simulink model "GVCU_HIL_simscape"  (R2026a)
settings: Solver=ode3  StartTime=0  StopTime=10  FixedStep=0.001
model workspace (MAT data in the model file):
  CANoelibParameters : object (value not decoded)
values from neighbouring files (symbols this model uses):
  acc_pedal_data = pedal_data.accelerator_pedal_position_t0    [Init_Simscape_main.m]
  acc_pedal_time = pedal_data.t0    [Init_Simscape_main.m]
  brk_pedal_data = brake_pedal_data.shared_brakes_drvrBrkPedlPerc_t0    [Init_Simscape_main.m]
  brk_pedal_time = brake_pedal_data.t0    [Init_Simscape_main.m]
  cycle_len = zeros(1, num_cycles)    [Init_Simscape_main.m]
  cycle_speed_matrix = zeros(max_cycle_len, num_cycles)    [Init_Simscape_main.m]
  cycle_time_matrix = zeros(max_cycle_len, num_cycles)    [Init_Simscape_main.m]
  veh_speed_data = speed_data.shared_dynamicsVso_vehVelLgt_t0    [Init_Simscape_main.m]
  veh_speed_time = speed_data.t0    [Init_Simscape_main.m]
undefined symbols (not defined in the file or in its folder): Active, aero, AuxActive, bat, brake, config, environment, FL, FL_prs_voltage, FR, FR_prs_voltage, front, pos, powertrain, rear, RL, RL_prs_voltage, RR, RR_prs_voltage, tir, veh, VGetRawValueFlag, Voltage, VT2816_1_Ch1, VT2816_1_Ch2, VT2816_1_Ch3, VT2816_1_Ch4, VT2816_3_Ch13, VT2816_3_Ch14, VT7101_1_Out2, VTS, X, Y, Z
libraries: sm_lib x358, fl_lib x272, nesl_utility x193, canoelib x127, sdl_lib x36, autolibsharedcoupling x21, autolibcoupling x9, slpidlib x7, simulink x3, autolibshareddiff x3, autolibshared x3, autolibutils x1
(part 2 of 17)

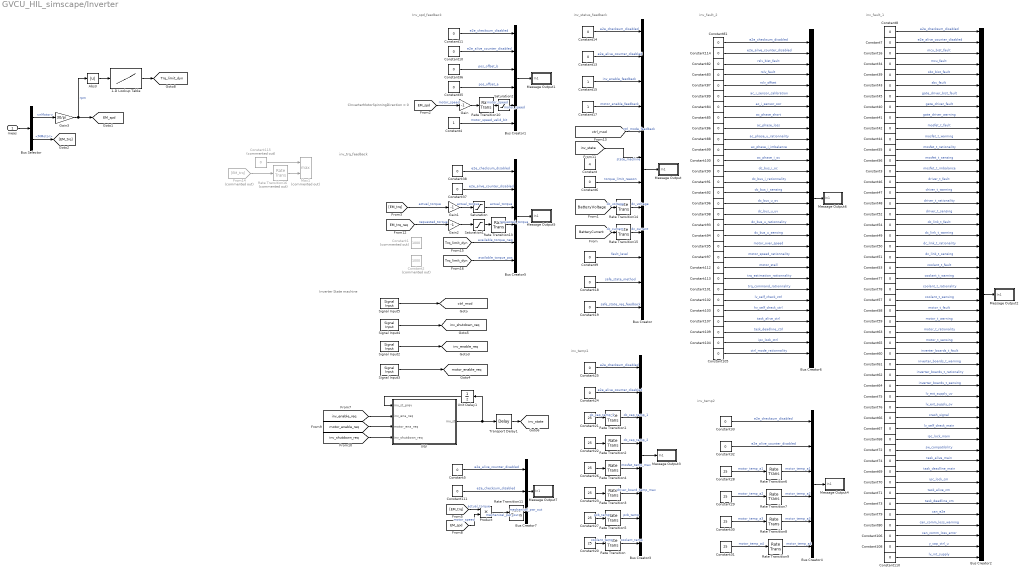
== system GVCU_HIL_simscape/Inverter ==
  note: CInverterMotorSpinningDirection = 0
  note: inv_fault_2
  note: inv_fault_1
  note: inv_trq_feedback
  note: Inv_spd_feedback
  note: Inverter State machine
  note: inv_temp2
  note: inv_temp1
  note: inv_status_feedback
  meas : Inport
  1-D Lookup Table : Lookup_n-D  NumberOfTableDimensions=1  BreakpointsForDimension1=[0, 2000, 3000, 4000, 5000, 6000]  Table=[825, 825, 700, 500, 500, 300]  ExtrapMethod=Clip  UseLastTableValue=on  InternalRulePriority=Speed  RndMeth=Simplest
  Abs3 : Abs  SaturateOnIntegerOverflow=off
  Bus Creator : BusCreator  Inputs=12
  Bus Creator1 : BusCreator  Inputs=6
  Bus Creator2 : BusCreator  Inputs=50
  Bus Creator3 : BusCreator  Inputs=8
  Bus Creator4 : BusCreator  Inputs=6
  Bus Creator5 : BusCreator  Inputs=6
  Bus Creator6 : BusCreator  Inputs=30
  Bus Creator7 : BusCreator  Inputs=3
  Bus Selector : BusSelector  OutputSignals=powertrain.nMotor,powertrain.MMotor
  Constant : Constant  Value=4
  Constant1 : Constant  Commented=on  Value=1000
  Constant{3,5..11,13..14,16,18..19,24..25,32..114} (98 alike) : Constant  Value=0
  Constant115 : Constant  Commented=on  Value=0
  Constant15 : Constant
  Constant17 : Constant
  Constant2 : Constant  Commented=on  Value=1000
  Constant20 : Constant  Value=25  OutDataTypeStr=uint8
  Constant21 : Constant  Value=25  OutDataTypeStr=uint8
  Constant{22..23,26..31} (8 alike) : Constant  Value=25
  Constant4 : Constant
  From14 : From  Commented=on  GotoTag=EM_trq  TagVisibility=global
  Gain : Gain  Gain=-1
  Gain1 : Gain  Gain=-1
  Gain2 : Gain  Gain=-1
  Gain3 : Gain  Gain=30/pi
  INV : MATLAB Function  TreatAsAtomicUnit=on
  Max1 : MinMax  Commented=on  Function=max  Inputs=2
  Message Output : Subsystem  AncestorBlock=canoelib/CANoe I//O/Message Output  mask(Signal Output Module){dbName=inverter_bus, nodeName=INV, msgName=inv_status_feedback, inputType=Bus Signal, rawValue=Default}
      mask prompts: dbName "Database name"; nodeName "Node name"; msgName "Message name"; inputType "Input type"; rawValue "Raw value"
      mask help: Output module for all signals of a databasemessage provided by the CANoe interaction layer. Double click the block for configuration.
      settings: AttributesFormatString=%<msgName>  CopyFcn=set_param(gcb, 'AttributesFormatString', '%<msgName>');  OpenFcn=MessageOutputBlock
      mask Help: For detailed information please refer to the CANoe online help 'MATLAB Integration Package » CANoe I/O Library'.
      mask TypeOptions inputType: Vector | Bus Signal
      mask TypeOptions rawValue: Default | Physical value | Raw value
      mask Display:
      | image(imread('MatlabBlock.png'))
      | disp('CANoe')
  Message Output1 : Subsystem  AncestorBlock=canoelib/CANoe I//O/Message Output  mask(Signal Output Module){dbName=inverter_bus, nodeName=INV, msgName=inv_spd_feedback, inputType=Bus Signal, rawValue=Default}
      mask prompts: dbName "Database name"; nodeName "Node name"; msgName "Message name"; inputType "Input type"; rawValue "Raw value"
      mask help: Output module for all signals of a databasemessage provided by the CANoe interaction layer. Double click the block for configuration.
      settings: AttributesFormatString=%<msgName>  CopyFcn=set_param(gcb, 'AttributesFormatString', '%<msgName>');  OpenFcn=MessageOutputBlock
      mask Help: For detailed information please refer to the CANoe online help 'MATLAB Integration Package » CANoe I/O Library'.
      mask TypeOptions inputType: Vector | Bus Signal
      mask TypeOptions rawValue: Default | Physical value | Raw value
      mask Display:
      | image(imread('MatlabBlock.png'))
      | disp('CANoe')
  Message Output2 : Subsystem  AncestorBlock=canoelib/CANoe I//O/Message Output  mask(Signal Output Module){dbName=inverter_bus, nodeName=INV, msgName=inv_fault_1, inputType=Bus Signal, rawValue=Default}
      mask prompts: dbName "Database name"; nodeName "Node name"; msgName "Message name"; inputType "Input type"; rawValue "Raw value"
      mask help: Output module for all signals of a databasemessage provided by the CANoe interaction layer. Double click the block for configuration.
      settings: AttributesFormatString=inv_fault_1  CopyFcn=set_param(gcb, 'AttributesFormatString', '%<msgName>');  OpenFcn=MessageOutputBlock
      mask Help: For detailed information please refer to the CANoe online help 'MATLAB Integration Package » CANoe I/O Library'.
      mask TypeOptions inputType: Vector | Bus Signal
      mask TypeOptions rawValue: Default | Physical value | Raw value
      mask Display:
      | image(imread('MatlabBlock.png'))
      | disp('CANoe')
  Message Output3 : Subsystem  AncestorBlock=canoelib/CANoe I//O/Message Output  mask(Signal Output Module){dbName=inverter_bus, nodeName=INV, msgName=inv_temperature_1, inputType=Bus Signal, rawValue=Default}
      mask prompts: dbName "Database name"; nodeName "Node name"; msgName "Message name"; inputType "Input type"; rawValue "Raw value"
      mask help: Output module for all signals of a databasemessage provided by the CANoe interaction layer. Double click the block for configuration.
      settings: AttributesFormatString=%<msgName>  CopyFcn=set_param(gcb, 'AttributesFormatString', '%<msgName>');  OpenFcn=MessageOutputBlock
      mask Help: For detailed information please refer to the CANoe online help 'MATLAB Integration Package » CANoe I/O Library'.
      mask TypeOptions inputType: Vector | Bus Signal
      mask TypeOptions rawValue: Default | Physical value | Raw value
      mask Display:
      | image(imread('MatlabBlock.png'))
      | disp('CANoe')
  Message Output4 : Subsystem  AncestorBlock=canoelib/CANoe I//O/Message Output  mask(Signal Output Module){dbName=inverter_bus, nodeName=INV, msgName=inv_temperature_2, inputType=Bus Signal, rawValue=Default}
      mask prompts: dbName "Database name"; nodeName "Node name"; msgName "Message name"; inputType "Input type"; rawValue "Raw value"
      mask help: Output module for all signals of a databasemessage provided by the CANoe interaction layer. Double click the block for configuration.
      settings: AttributesFormatString=%<msgName>  CopyFcn=set_param(gcb, 'AttributesFormatString', '%<msgName>');  OpenFcn=MessageOutputBlock
      mask Help: For detailed information please refer to the CANoe online help 'MATLAB Integration Package » CANoe I/O Library'.
      mask TypeOptions inputType: Vector | Bus Signal
      mask TypeOptions rawValue: Default | Physical value | Raw value
      mask Display:
      | image(imread('MatlabBlock.png'))
      | disp('CANoe')
  Message Output5 : Subsystem  AncestorBlock=canoelib/CANoe I//O/Message Output  mask(Signal Output Module){dbName=inverter_bus, nodeName=INV, msgName=inv_trq_feedback, inputType=Bus Signal, rawValue=Default}
      mask prompts: dbName "Database name"; nodeName "Node name"; msgName "Message name"; inputType "Input type"; rawValue "Raw value"
      mask help: Output module for all signals of a databasemessage provided by the CANoe interaction layer. Double click the block for configuration.
      settings: AttributesFormatString=%<msgName>  CopyFcn=set_param(gcb, 'AttributesFormatString', '%<msgName>');  OpenFcn=MessageOutputBlock
      mask Help: For detailed information please refer to the CANoe online help 'MATLAB Integration Package » CANoe I/O Library'.
      mask TypeOptions inputType: Vector | Bus Signal
      mask TypeOptions rawValue: Default | Physical value | Raw value
      mask Display:
      | image(imread('MatlabBlock.png'))
      | disp('CANoe')
  Message Output6 : Subsystem  AncestorBlock=canoelib/CANoe I//O/Message Output  mask(Signal Output Module){dbName=inverter_bus, nodeName=INV, msgName=inv_fault_2, inputType=Bus Signal, rawValue=Default}
      mask prompts: dbName "Database name"; nodeName "Node name"; msgName "Message name"; inputType "Input type"; rawValue "Raw value"
      mask help: Output module for all signals of a databasemessage provided by the CANoe interaction layer. Double click the block for configuration.
      settings: AttributesFormatString=%<msgName>  CopyFcn=set_param(gcb, 'AttributesFormatString', '%<msgName>');  OpenFcn=MessageOutputBlock
      mask Help: For detailed information please refer to the CANoe online help 'MATLAB Integration Package » CANoe I/O Library'.
      mask TypeOptions inputType: Vector | Bus Signal
      mask TypeOptions rawValue: Default | Physical value | Raw value
      mask Display:
      | image(imread('MatlabBlock.png'))
      | disp('CANoe')
  Message Output7 : Subsystem  AncestorBlock=canoelib/CANoe I//O/Message Output  mask(Signal Output Module){dbName=inverter_bus, nodeName=INV, msgName=inv_pwr_feedback, inputType=Bus Signal, rawValue=Default}
      mask prompts: dbName "Database name"; nodeName "Node name"; msgName "Message name"; inputType "Input type"; rawValue "Raw value"
      mask help: Output module for all signals of a databasemessage provided by the CANoe interaction layer. Double click the block for configuration.
      settings: AttributesFormatString=%<msgName>  CopyFcn=set_param(gcb, 'AttributesFormatString', '%<msgName>');  OpenFcn=MessageOutputBlock
      mask Help: For detailed information please refer to the CANoe online help 'MATLAB Integration Package » CANoe I/O Library'.
      mask TypeOptions inputType: Vector | Bus Signal
      mask TypeOptions rawValue: Default | Physical value | Raw value
      mask Display:
      | image(imread('MatlabBlock.png'))
      | disp('CANoe')
  Product : Product
  Rate Transition{,1..9} (10 alike) : RateTransition  OutPortSampleTime=1
  Rate Transition10 : RateTransition  OutPortSampleTime=0.004
  Rate Transition11 : RateTransition  OutPortSampleTime=0.004
  Rate Transition13 : RateTransition  OutPortSampleTime=0.004
  Rate Transition14 : RateTransition  OutPortSampleTime=0.1
  Rate Transition15 : RateTransition  OutPortSampleTime=0.1
  Rate Transition16 : RateTransition  Commented=on  OutPortSampleTime=0.005
  Saturation : Saturate  UpperLimit=2047  LowerLimit=-2048
  Saturation1 : Saturate  UpperLimit=2047  LowerLimit=-2048
  Saturation2 : Saturate  UpperLimit=16383  LowerLimit=-16384
  Signal Input2 : canoelib/CANoe I//O/Signal Input  dbName=inverter_bus  nodeName=GVCU  msgName=inv_cmd  sigName=inv_enable_req  editSampleTime=0  rawValue=Default  dataType=Default  dataTypeDB=boolean  hasEncoding=off
      settings: AttributesFormatString=%<sigName>  SourceProductName=Vector CANoe
  Signal Input3 : canoelib/CANoe I//O/Signal Input  dbName=inverter_bus  nodeName=GVCU  msgName=inv_cmd  sigName=motor_enable_req  editSampleTime=0  rawValue=Default  dataType=Default  dataTypeDB=boolean  hasEncoding=off
      settings: AttributesFormatString=%<sigName>  SourceProductName=Vector CANoe
  Signal Input4 : canoelib/CANoe I//O/Signal Input  dbName=inverter_bus  nodeName=GVCU  msgName=inv_cmd  sigName=shutdown_req  editSampleTime=0  rawValue=Default  dataType=Default  dataTypeDB=boolean  hasEncoding=off
      settings: AttributesFormatString=%<sigName>  SourceProductName=Vector CANoe
  Signal Input5 : canoelib/CANoe I//O/Signal Input  dbName=inverter_bus  nodeName=GVCU  msgName=inv_cmd  sigName=ctrl_mode_req  editSampleTime=0  rawValue=Default  dataType=Default  dataTypeDB=uint8  hasEncoding=off
      settings: AttributesFormatString=%<sigName>  SourceProductName=Vector CANoe
  Transport Delay1 : TransportDelay
  Unit Delay1 : UnitDelay  SampleTime=-1
  tag scope: EM_spd=global, Trq_limit_dyn=global, ctrl_mod=global, inv_enable_req=global, inv_shutdown_req=global, inv_state=global, motor_enable_req=global
  wires:
  [Trq_limit_dyn] -> Bus Creator5/5  "available_torque_neg"
  [Trq_limit_dyn] -> Bus Creator5/6  "available_torque_pos"
  [EM_trq] -> Gain1/1  "actual_torque"
  Constant4/1 -> Bus Creator1/6  "motor_speed_valid_bit"
  Rate Transition10/1 -> Saturation2/1  "motor_speed"
  Constant6/1 -> Bus Creator/7  "torque_limit_reason"
  Constant10/1 -> Bus Creator1/2  "e2e_alive_counter_disabled"
  Constant11/1 -> Bus Creator1/1  "e2e_checksum_disabled"
  Rate Transition15/1 -> Bus Creator/9  "dc_current"
  Rate Transition14/1 -> Bus Creator/8  "dc_voltage"
  Rate Transition/1 -> Bus Creator3/8  "coolant_temp"
  Rate Transition1/1 -> Bus Creator3/3  "dc_cap_temp_1"
  Rate Transition3/1 -> Bus Creator3/6  "driver_board_temp_max"
  Rate Transition2/1 -> Bus Creator3/4  "dc_cap_temp_2"
  Constant24/1 -> Bus Creator3/2  "e2e_alive_counter_disabled"
  Constant25/1 -> Bus Creator3/1  "e2e_checksum_disabled"
  Rate Transition4/1 -> Bus Creator3/5  "mosfet_temp_max"
  Rate Transition5/1 -> Bus Creator3/7  "pcb_temp"
  Rate Transition6/1 -> Bus Creator4/3  "motor_temp_a1"
  Rate Transition7/1 -> Bus Creator4/4  "motor_temp_a2"
  Rate Transition8/1 -> Bus Creator4/5  "motor_temp_a3"
  Rate Transition9/1 -> Bus Creator4/6  "motor_temp_a4"
  Constant32/1 -> Bus Creator4/2  "e2e_alive_counter_disabled"
  Constant33/1 -> Bus Creator4/1  "e2e_checksum_disabled"
  Signal Input2/1 -> [inv_enable_req]
  Signal Input3/1 -> [motor_enable_req]
  Signal Input4/1 -> [inv_shutdown_req]
  [inv_enable_req] -> INV/2(inv_ena_req)
  [motor_enable_req] -> INV/3(motor_ena_req)
  [inv_shutdown_req] -> INV/4(inv_shutdown_req)
  INV/1(inv_st) -> Unit Delay1/1, Transport Delay1/1
  Transport Delay1/1 -> [inv_state]
  Unit Delay1/1 -> INV/1(inv_st_prev)
  Bus Creator/1 -> Message Output/1(In1)
  Bus Creator3/1 -> Message Output3/1(In1)
  Bus Creator4/1 -> Message Output4/1(In1)
  Constant35/1 -> Bus Creator1/4  "pos_offset_a"
  Constant36/1 -> Bus Creator1/3  "pos_offset_b"
  Bus Creator1/1 -> Message Output1/1(In1)
  Constant37/1 -> Bus Creator5/2  "e2e_alive_counter_disabled"
  Constant38/1 -> Bus Creator5/1  "e2e_checksum_disabled"
  Rate Transition13/1 -> Bus Creator5/4  "requested_torque"
  Bus Creator5/1 -> Message Output5/1(In1)
  Constant18/1 -> Bus Creator/11  "safe_state_method"
  Constant19/1 -> Bus Creator/12  "safe_state_req_feedback"
  Constant14/1 -> Bus Creator/1  "e2e_checksum_disabled"
  Constant13/1 -> Bus Creator/2  "e2e_alive_counter_disabled"
  [inv_state] -> Bus Creator/6  "state_machine"
  [ctrl_mod] -> Bus Creator/5  "ctrl_mode_feedback"
  Constant17/1 -> Bus Creator/4  "motor_enable_feedback"
  Constant15/1 -> Bus Creator/3  "inv_enable_feedback"
  Constant9/1 -> Bus Creator/10  "fault_level"
  Constant7/1 -> Bus Creator2/2  "e2e_alive_counter_disabled"
  Constant8/1 -> Bus Creator2/1  "e2e_checksum_disabled"
  Constant16/1 -> Bus Creator2/3  "mcu_bist_fault"
  Constant40/1 -> Bus Creator2/8  "gate_driver_fault"
  Constant45/1 -> Bus Creator2/7  "gate_driver_bist_fault"
  Constant54/1 -> Bus Creator2/19  "dc_link_t_fault"
  Constant46/1 -> Bus Creator2/15  "driver_t_fault"
  Constant56/1 -> Bus Creator2/13  "mosfet_t_sensing"
  Constant55/1 -> Bus Creator2/12  "mosfet_t_rationality"
  Constant34/1 -> Bus Creator2/4  "mcu_fault"
  Constant39/1 -> Bus Creator2/5  "sbc_bist_fault"
  Constant43/1 -> Bus Creator2/6  "sbc_fault"
  Constant41/1 -> Bus Creator2/9  "gate_driver_warning"
  Constant42/1 -> Bus Creator2/10  "mosfet_t_fault"
  Constant44/1 -> Bus Creator2/11  "mosfet_t_warning"
  Constant47/1 -> Bus Creator2/16  "driver_t_warning"
  Constant48/1 -> Bus Creator2/17  "driver_t_rationality"
  Constant52/1 -> Bus Creator2/18  "driver_t_sensing"
  Constant49/1 -> Bus Creator2/20  "dc_link_t_warning"
  Constant50/1 -> Bus Creator2/21  "dc_link_t_rationality"
  Constant51/1 -> Bus Creator2/22  "dc_link_t_sensing"
  Constant53/1 -> Bus Creator2/23  "coolant_t_fault"
  Constant77/1 -> Bus Creator2/24  "coolant_t_warning"
  Constant78/1 -> Bus Creator2/25  "coolant_t_rationality"
  Constant57/1 -> Bus Creator2/26  "coolant_t_sensing"
  Constant58/1 -> Bus Creator2/27  "motor_t_fault"
  Constant59/1 -> Bus Creator2/28  "motor_t_warning"
  Constant63/1 -> Bus Creator2/29  "motor_t_rationality"
  Constant65/1 -> Bus Creator2/30  "motor_t_sensing"
  Constant60/1 -> Bus Creator2/31  "inverter_boards_t_fault"
  Constant61/1 -> Bus Creator2/32  "inverter_boards_t_warning"
  Constant62/1 -> Bus Creator2/33  "inverter_boards_t_rationality"
  Constant64/1 -> Bus Creator2/34  "inverter_boards_t_sensing"
  Constant75/1 -> Bus Creator2/35  "lv_ext_supply_uv"
  Constant76/1 -> Bus Creator2/36  "lv_ext_supply_ov"
  Constant66/1 -> Bus Creator2/37  "crash_signal"
  Constant67/1 -> Bus Creator2/38  "lv_self_check_main"
  Constant68/1 -> Bus Creator2/39  "ipc_lock_main"
  Constant72/1 -> Bus Creator2/40  "sw_compatibility"
  Constant74/1 -> Bus Creator2/41  "task_alive_main"
  Constant69/1 -> Bus Creator2/42  "task_deadline_main"
  Constant70/1 -> Bus Creator2/43  "ipc_lock_cm"
  Constant71/1 -> Bus Creator2/44  "task_alive_cm"
  Constant73/1 -> Bus Creator2/45  "task_deadline_cm"
  Constant80/1 -> Bus Creator2/47  "can_comm_loss_warning"
  Constant79/1 -> Bus Creator2/46  "can_e2e"
  Bus Creator2/1 -> Message Output2/1(In1)
  Constant86/1 -> Bus Creator6/9  "ac_phase_loss"
  Constant85/1 -> Bus Creator6/8  "ac_phase_short"
  Constant84/1 -> Bus Creator6/7  "ac_i_sensor_oor"
  Constant89/1 -> Bus Creator6/6  "ac_i_sensor_calibration"
  Constant83/1 -> Bus Creator6/4  "rslv_fault"
  Constant87/1 -> Bus Creator6/5  "rslv_offset"
  Constant82/1 -> Bus Creator6/3  "rslv_bist_fault"
  Constant81/1 -> Bus Creator6/1  "e2e_checksum_disabled"
  Constant114/1 -> Bus Creator6/2  "e2e_alive_counter_disabled"
  Constant88/1 -> Bus Creator6/10  "ac_phase_u_rationnality"
  Constant99/1 -> Bus Creator6/11  "ac_phase_i_imbalance"
  Constant100/1 -> Bus Creator6/12  "ac_phase_i_oc"
  Constant90/1 -> Bus Creator6/13  "dc_bus_i_oc"
  Constant91/1 -> Bus Creator6/14  "dc_bus_i_rationnality"
  Constant92/1 -> Bus Creator6/15  "dc_bus_i_sensing"
  Constant96/1 -> Bus Creator6/16  "dc_bus_u_ov"
  Constant98/1 -> Bus Creator6/17  "dc_bus_u_uv"
  Constant93/1 -> Bus Creator6/18  "dc_bus_u_rationnality"
  Constant94/1 -> Bus Creator6/19  "dc_bus_u_sensing"
  Constant95/1 -> Bus Creator6/20  "motor_over_speed"
  Constant97/1 -> Bus Creator6/21  "motor_speed_rationnality"
  Constant112/1 -> Bus Creator6/22  "motor_stall"
  Constant113/1 -> Bus Creator6/23  "trq_estimation_rationnality"
  Constant101/1 -> Bus Creator6/24  "trq_command_rationnality"
  Constant102/1 -> Bus Creator6/25  "lv_self_check_ctrl"
  Constant103/1 -> Bus Creator6/26  "hv_self_check_ctrl"
  Constant107/1 -> Bus Creator6/27  "task_alive_ctrl"
  Constant109/1 -> Bus Creator6/28  "task_deadline_ctrl"
  Constant104/1 -> Bus Creator6/29  "ipc_lock_ctrl"
  Constant105/1 -> Bus Creator6/30  "ctrl_mode_rationnality"
  Bus Creator6/1 -> Message Output6/1(In1)
  Constant106/1 -> Bus Creator2/48  "can_comm_loss_error"
  Constant108/1 -> Bus Creator2/49  "y_cap_ctrl_u"
  Constant110/1 -> Bus Creator2/50  "lv_int_supply"
  Constant20/1 -> Rate Transition/1  "coolant_temp"
  Constant21/1 -> Rate Transition1/1  "dc_cap_temp_1"
  Constant22/1 -> Rate Transition2/1
  Constant23/1 -> Rate Transition3/1
  Constant26/1 -> Rate Transition4/1
  Constant27/1 -> Rate Transition5/1  "pcb_temp"
  Constant28/1 -> Rate Transition6/1  "motor_temp_a1"
  Constant29/1 -> Rate Transition7/1  "motor_temp_a2"
  Constant30/1 -> Rate Transition8/1  "motor_temp_a3"
  Constant31/1 -> Rate Transition9/1  "motor_temp_a4"
  [EM_trq] -> Product/1  "actual_torque"
  [EM_spd] -> Product/2  "motor_speed"
  Rate Transition11/1 -> Bus Creator7/3  "mechanical_pwr_out"
  Constant111/1 -> Bus Creator7/2  "e2e_checksum_disabled"
  Constant5/1 -> Bus Creator7/1  "e2e_alive_counter_disabled"
  Bus Creator7/1 -> Message Output7/1(In1)
  [EM_spd] -> Gain/1  "motor_speed"
  [EM_trq_req] -> Gain2/1  "requested_torque"
  Product/1 -> Rate Transition11/1  "mechanical_pwr_out"
  [BatteryVoltage] -> Rate Transition14/1  "dc_voltage"
  [BatteryCurrent] -> Rate Transition15/1  "dc_current"
  Signal Input5/1 -> [ctrl_mod]
  Constant3/1 -> Bus Creator2/14  "mosfet_t_imbalance"
  Gain/1 -> Rate Transition10/1
  Gain1/1 -> Saturation/1  "actual_torque"
  Gain2/1 -> Saturation1/1
  Constant115/1 -> Max1/1
  Rate Transition16/1 -> Max1/2
  From14/1 -> Rate Transition16/1
  Saturation/1 -> Bus Creator5/3  "actual_torque"
  Saturation1/1 -> Rate Transition13/1
  Saturation2/1 -> Bus Creator1/5  "motor_speed"
  meas/1 -> Bus Selector/1
  Bus Selector/2 -> [EM_trq]  "<MMotor>"
  Bus Selector/1 -> Gain3/1  "<nMotor>"
  1-D Lookup Table/1 -> [Trq_limit_dyn]
  Gain3/1 -> Abs3/1, [EM_spd]  "rpm"
  Abs3/1 -> 1-D Lookup Table/1

== system GVCU_HIL_simscape/Model_observation ==
  note: Vehicle model
  note: Powertrain model
  note: Front axle model
  note: Driver model
  note: AWD Powertrain model
  From10 : From  Commented=on  GotoTag=FR_R_Spd  TagVisibility=global
  From11 : From  Commented=on  GotoTag=FR_G_Spd  TagVisibility=global
  From16 : From  Commented=on  GotoTag=Axl_centre_Spd  TagVisibility=global
  From6 : From  Commented=on  GotoTag=FL_R_Spd  TagVisibility=global
  From7 : From  Commented=on  GotoTag=FL_G_Spd  TagVisibility=global
  System Variable Output : canoelib/CANoe I//O/System Variable Output  nsName=Checker_Simulink  sysVarName=ModelVel  arrayIndex=-1  rawValue=Default  dataType=Default  dataTypeDB=double  hasEncoding=off  dataTypeCANoe=Get from CANoe
      settings: AttributesFormatString=%<nsName>::%<sysVarName>  SourceProductName=Vector CANoe
  System Variable Output1 : canoelib/CANoe I//O/System Variable Output  Commented=on  nsName=AWD_Powertrain  sysVarName=FR_R_Spd  arrayIndex=-1  rawValue=Default  dataType=Default  dataTypeDB=int32  hasEncoding=off  dataTypeCANoe=Get from CANoe
      settings: AttributesFormatString=%<nsName>::%<sysVarName>  SourceProductName=Vector CANoe
  System Variable Output10 : canoelib/CANoe I//O/System Variable Output  Commented=on  nsName=AWD_Powertrain  sysVarName=FL_G_Spd  arrayIndex=-1  rawValue=Default  dataType=Default  dataTypeDB=int32  hasEncoding=off  dataTypeCANoe=Get from CANoe
      settings: AttributesFormatString=%<nsName>::%<sysVarName>  SourceProductName=Vector CANoe
  System Variable Output11 : canoelib/CANoe I//O/System Variable Output  nsName=Checker_Simulink  sysVarName=brake_switch  arrayIndex=-1  rawValue=Default  dataType=Default  dataTypeDB=int32  hasEncoding=off  dataTypeCANoe=Get from CANoe
      settings: AttributesFormatString=%<nsName>::%<sysVarName>  SourceProductName=Vector CANoe
  System Variable Output12 : canoelib/CANoe I//O/System Variable Output  nsName=Checker_Simulink  sysVarName=Acc_Cmd  arrayIndex=-1  rawValue=Default  dataType=Default  dataTypeDB=double  hasEncoding=off  dataTypeCANoe=Get from CANoe
      settings: AttributesFormatString=%<nsName>::%<sysVarName>  SourceProductName=Vector CANoe
  System Variable Output13 : canoelib/CANoe I//O/System Variable Output  nsName=Checker_Simulink  sysVarName=VelRef_drv_mod_in  arrayIndex=-1  rawValue=Default  dataType=Default  dataTypeDB=double  hasEncoding=off  dataTypeCANoe=Get from CANoe
      settings: AttributesFormatString=%<nsName>::%<sysVarName>  SourceProductName=Vector CANoe
  System Variable Output14 : canoelib/CANoe I//O/System Variable Output  nsName=AWD_Powertrain  sysVarName=Axl_front_Spd  arrayIndex=-1  rawValue=Default  dataType=Default  dataTypeDB=int32  hasEncoding=off  dataTypeCANoe=Get from CANoe
      settings: AttributesFormatString=%<nsName>::%<sysVarName>  SourceProductName=Vector CANoe
  System Variable Output15 : canoelib/CANoe I//O/System Variable Output  Commented=on  nsName=AWD_Powertrain  sysVarName=Axl_centre_Spd  arrayIndex=-1  rawValue=Default  dataType=Default  dataTypeDB=int32  hasEncoding=off  dataTypeCANoe=Get from CANoe
      settings: AttributesFormatString=%<nsName>::%<sysVarName>  SourceProductName=Vector CANoe
  System Variable Output16 : canoelib/CANoe I//O/System Variable Output  nsName=AWD_Powertrain  sysVarName=FR_clu_prs  arrayIndex=-1  rawValue=Default  dataType=Default  dataTypeDB=int32  hasEncoding=off  dataTypeCANoe=Get from CANoe
      settings: AttributesFormatString=%<nsName>::%<sysVarName>  SourceProductName=Vector CANoe
  System Variable Output17 : canoelib/CANoe I//O/System Variable Output  nsName=AWD_Powertrain  sysVarName=Split_tors_FR  arrayIndex=-1  rawValue=Default  dataType=Default  dataTypeDB=int32  hasEncoding=off  dataTypeCANoe=Get from CANoe
      settings: AttributesFormatString=%<nsName>::%<sysVarName>  SourceProductName=Vector CANoe
  System Variable Output18 : canoelib/CANoe I//O/System Variable Output  nsName=AWD_Powertrain  sysVarName=Split_tors_FL  arrayIndex=-1  rawValue=Default  dataType=Default  dataTypeDB=int32  hasEncoding=off  dataTypeCANoe=Get from CANoe
      settings: AttributesFormatString=%<nsName>::%<sysVarName>  SourceProductName=Vector CANoe
  System Variable Output19 : canoelib/CANoe I//O/System Variable Output  nsName=Checker_Simulink  sysVarName=EM_trq_cmd  arrayIndex=-1  rawValue=Default  dataType=Default  dataTypeDB=int32  hasEncoding=off  dataTypeCANoe=Get from CANoe
      settings: AttributesFormatString=%<nsName>::%<sysVarName>  SourceProductName=Vector CANoe
  System Variable Output2 : canoelib/CANoe I//O/System Variable Output  Commented=on  nsName=AWD_Powertrain  sysVarName=FR_G_Spd  arrayIndex=-1  rawValue=Default  dataType=Default  dataTypeDB=int32  hasEncoding=off  dataTypeCANoe=Get from CANoe
      settings: AttributesFormatString=%<nsName>::%<sysVarName>  SourceProductName=Vector CANoe
  System Variable Output20 : canoelib/CANoe I//O/System Variable Output  nsName=Checker_Simulink  sysVarName=EM_trq_req_received  arrayIndex=-1  rawValue=Default  dataType=Default  dataTypeDB=int32  hasEncoding=off  dataTypeCANoe=Get from CANoe
      settings: AttributesFormatString=%<nsName>::%<sysVarName>  SourceProductName=Vector CANoe
  System Variable Output21 : canoelib/CANoe I//O/System Variable Output  nsName=Checker_Simulink  sysVarName=Brake_prs_front  arrayIndex=-1  rawValue=Default  dataType=Default  dataTypeDB=int32  hasEncoding=off  dataTypeCANoe=Get from CANoe
      settings: AttributesFormatString=%<nsName>::%<sysVarName>  SourceProductName=Vector CANoe
  System Variable Output22 : canoelib/CANoe I//O/System Variable Output  nsName=Checker_Simulink  sysVarName=Brake_prs_rear  arrayIndex=-1  rawValue=Default  dataType=Default  dataTypeDB=int32  hasEncoding=off  dataTypeCANoe=Get from CANoe
      settings: AttributesFormatString=%<nsName>::%<sysVarName>  SourceProductName=Vector CANoe
  System Variable Output23 : canoelib/CANoe I//O/System Variable Output  nsName=AWD_Powertrain  sysVarName=FL_clu_prs  arrayIndex=-1  rawValue=Default  dataType=Default  dataTypeDB=int32  hasEncoding=off  dataTypeCANoe=Get from CANoe
      settings: AttributesFormatString=%<nsName>::%<sysVarName>  SourceProductName=Vector CANoe
  System Variable Output24 : canoelib/CANoe I//O/System Variable Output  nsName=AWD_Powertrain  sysVarName=RR_clu_prs  arrayIndex=-1  rawValue=Default  dataType=Default  dataTypeDB=int32  hasEncoding=off  dataTypeCANoe=Get from CANoe
      settings: AttributesFormatString=%<nsName>::%<sysVarName>  SourceProductName=Vector CANoe
  System Variable Output25 : canoelib/CANoe I//O/System Variable Output  nsName=AWD_Powertrain  sysVarName=RL_clu_prs  arrayIndex=-1  rawValue=Default  dataType=Default  dataTypeDB=int32  hasEncoding=off  dataTypeCANoe=Get from CANoe
      settings: AttributesFormatString=%<nsName>::%<sysVarName>  SourceProductName=Vector CANoe
  System Variable Output26 : canoelib/CANoe I//O/System Variable Output  nsName=Checker_Simulink  sysVarName=PID_EM_error  arrayIndex=-1  rawValue=Default  dataType=Default  dataTypeDB=int32  hasEncoding=off  dataTypeCANoe=Get from CANoe
      settings: AttributesFormatString=%<nsName>::%<sysVarName>  SourceProductName=Vector CANoe
  System Variable Output27 : canoelib/CANoe I//O/System Variable Output  nsName=Checker_Simulink  sysVarName=DecCmd  arrayIndex=-1  rawValue=Default  dataType=Default  dataTypeDB=int32  hasEncoding=off  dataTypeCANoe=Get from CANoe
      settings: AttributesFormatString=%<nsName>::%<sysVarName>  SourceProductName=Vector CANoe
  System Variable Output3 : canoelib/CANoe I//O/System Variable Output  nsName=Checker_Simulink  sysVarName=Force_front_wheel  arrayIndex=-1  rawValue=Default  dataType=Default  dataTypeDB=int32  hasEncoding=off  dataTypeCANoe=Get from CANoe
      settings: AttributesFormatString=%<nsName>::%<sysVarName>  SourceProductName=Vector CANoe
  System Variable Output4 : canoelib/CANoe I//O/System Variable Output  nsName=Checker_Simulink  sysVarName=Force_rear_wheel  arrayIndex=-1  rawValue=Default  dataType=Default  dataTypeDB=int32  hasEncoding=off  dataTypeCANoe=Get from CANoe
      settings: AttributesFormatString=%<nsName>::%<sysVarName>  SourceProductName=Vector CANoe
  System Variable Output5 : canoelib/CANoe I//O/System Variable Output  nsName=Checker_Simulink  sysVarName=street_steepness  arrayIndex=-1  rawValue=Default  dataType=Default  dataTypeDB=int32  hasEncoding=off  dataTypeCANoe=Get from CANoe
      settings: AttributesFormatString=%<nsName>::%<sysVarName>  SourceProductName=Vector CANoe
  System Variable Output6 : canoelib/CANoe I//O/System Variable Output  nsName=Checker_Simulink  sysVarName=Force_wind  arrayIndex=-1  rawValue=Default  dataType=Default  dataTypeDB=int32  hasEncoding=off  dataTypeCANoe=Get from CANoe
      settings: AttributesFormatString=%<nsName>::%<sysVarName>  SourceProductName=Vector CANoe
  System Variable Output7 : canoelib/CANoe I//O/System Variable Output  nsName=Checker_Simulink  sysVarName=EM_trq  arrayIndex=-1  rawValue=Default  dataType=Default  dataTypeDB=int32  hasEncoding=off  dataTypeCANoe=Get from CANoe
      settings: AttributesFormatString=%<nsName>::%<sysVarName>  SourceProductName=Vector CANoe
  System Variable Output8 : canoelib/CANoe I//O/System Variable Output  nsName=Checker_Simulink  sysVarName=EM_Spd  arrayIndex=-1  rawValue=Default  dataType=Default  dataTypeDB=int32  hasEncoding=off  dataTypeCANoe=Get from CANoe
      settings: AttributesFormatString=%<nsName>::%<sysVarName>  SourceProductName=Vector CANoe
  System Variable Output9 : canoelib/CANoe I//O/System Variable Output  Commented=on  nsName=AWD_Powertrain  sysVarName=FL_R_Spd  arrayIndex=-1  rawValue=Default  dataType=Default  dataTypeDB=int32  hasEncoding=off  dataTypeCANoe=Get from CANoe
      settings: AttributesFormatString=%<nsName>::%<sysVarName>  SourceProductName=Vector CANoe
  wires:
  [EM_trq] -> System Variable Output7/1
  [EM_trq_cmd] -> System Variable Output19/1
  [Force_front_wheel] -> System Variable Output3/1
  [Force_wind] -> System Variable Output6/1
  [street_steepness] -> System Variable Output5/1
  [Force_rear_wheel] -> System Variable Output4/1
  [ModelVel] -> System Variable Output/1  "km/h"
  From6/1 -> System Variable Output9/1
  From7/1 -> System Variable Output10/1
  From10/1 -> System Variable Output1/1
  From11/1 -> System Variable Output2/1
  [brake_switch] -> System Variable Output11/1
  [AccCmd] -> System Variable Output12/1
  [VelRef_drv_mod_in] -> System Variable Output13/1
  [Axl_front_Spd] -> System Variable Output14/1
  From16/1 -> System Variable Output15/1
  [Split_tors_FR] -> System Variable Output17/1
  [Split_tors_FL] -> System Variable Output18/1
  [EM_spd] -> System Variable Output8/1
  [EM_trq_req] -> System Variable Output20/1
  [Brake_prs_front] -> System Variable Output21/1
  [Brake_prs_rear] -> System Variable Output22/1
  [FL_prs] -> System Variable Output23/1
  [FR_prs] -> System Variable Output16/1
  [RL_prs] -> System Variable Output25/1
  [RR_prs] -> System Variable Output24/1
  [PID_EM_error] -> System Variable Output26/1
  [DecCmd] -> System Variable Output27/1

== system GVCU_HIL_simscape/Powertrain (EV) ==
  1-D Lookup Table : Lookup_n-D  Commented=on  NumberOfTableDimensions=1  BreakpointsForDimension1=[0, 2000, 3000, 4000, 5000, 6000]  Table=[825, 825, 700, 500, 500, 300]  ExtrapMethod=Clip  UseLastTableValue=on  InternalRulePriority=Speed  RndMeth=Simplest
  AWD_Powertrain1 : Subsystem  Commented=on
  Abs3 : Abs  Commented=on  SaturateOnIntegerOverflow=off
  Compare To Constant : simulink/Logic and Bit Operations/Compare To Constant  relop=<  const=2  OutDataTypeStr=boolean
  Constant : Constant  Value=0
  Delay : Delay
  EM : Subsystem
      mask Display: image('$imagefile');
  FWD_ELEC_Powertrain : Subsystem  Commented=on
  FWD_ELEC_Powertrain_sorted : Subsystem  Commented=on
  From : From  Commented=on  GotoTag=EM_trq  TagVisibility=global
  Gain1 : Gain  Commented=on  Gain=30/pi
  Gain2 : Gain  Gain=pi/30
  Goto : Goto  Commented=on  GotoTag=EM_spd  TagVisibility=global
  Goto8 : Goto  Commented=on  GotoTag=Trq_limit_dyn  TagVisibility=global
  Memory1 : Memory  Commented=on  InheritSampleTime=on
  PID Speed Controller : Subsystem
  PID Speed Ctrl Mode : Subsystem  Commented=on  TreatAsAtomicUnit=on
  Rate Limiter : RateLimiter  RisingSlewLimit=100000  FallingSlewLimit=-100000  SampleTimeMode=inherited
  Signal Input1 : canoelib/CANoe I//O/Signal Input  dbName=inverter_bus  nodeName=GVCU  msgName=inv_motion_cmd  sigName=speed_req  editSampleTime=0  rawValue=Default  dataType=Default  dataTypeDB=uint16  hasEncoding=on
      settings: AttributesFormatString=%<sigName>  SourceProductName=Vector CANoe
  Signal Input2 : canoelib/CANoe I//O/Signal Input  dbName=inverter_bus  nodeName=GVCU  msgName=inv_motion_cmd  sigName=torque_req  editSampleTime=0  rawValue=Default  dataType=Default  dataTypeDB=uint16  hasEncoding=on
      settings: AttributesFormatString=%<sigName>  SourceProductName=Vector CANoe
  Signal Input4 : canoelib/CANoe I//O/Signal Input  dbName=inverter_bus  nodeName=GVCU  msgName=inv_cmd  sigName=ctrl_mode_req  editSampleTime=0  rawValue=Default  dataType=Default  dataTypeDB=uint8  hasEncoding=off
      settings: AttributesFormatString=%<sigName>  SourceProductName=Vector CANoe
  Switch2 : Switch  Criteria=u2 > Threshold  Threshold=1  SaturateOnIntegerOverflow=off  InputSameDT=off
  Terminator : Terminator
  EM_trq_out : Outport  VectorParamsAs1DForOutWhenUnconnected=off
  tag scope: EM_trq_cmd=global, EM_trq_req=global, PID_EM_error=global
  wires:
  EM/2(EMTrq) -> EM_trq_out/1
  EM/1(Info) -> Terminator/1  "EM"
  FWD_ELEC_Powertrain_sorted/2(Axl_Trq1) -> ?
  Gain1/1 -> Abs3/1, Goto/1  "rpm"
  FWD_ELEC_Powertrain_sorted/1(EM_Spd) -> PID Speed Controller/1(speed_feedback), EM/2(EMSpd), Gain1/1  "rad/s"
  Switch2/1 -> [EM_trq_cmd], EM/1(TrqCmd)
  Signal Input4/1 -> Compare To Constant/1, Switch2/2
  PID Speed Controller/2(Trq_cmd_elecMot) -> Switch2/1
  Signal Input2/1 -> PID Speed Controller/4(trq_req), [EM_trq_req]
  Signal Input1/1 -> Rate Limiter/1  "rpm"
  Gain2/1 -> PID Speed Controller/3(speed_req)  "rad/s"
  PID Speed Controller/1(PID_EM_error) -> [PID_EM_error]
  From/1 -> Memory1/1
  Memory1/1 -> PID Speed Ctrl Mode/4(trq_act)
  1-D Lookup Table/1 -> Goto8/1
  Abs3/1 -> 1-D Lookup Table/1
  [Trq_limit_dyn] -> Delay/1
  Rate Limiter/1 -> Gain2/1  "rpm"
  Constant/1 -> Switch2/3
  Compare To Constant/1 -> PID Speed Controller/5(reset)
  Delay/1 -> PID Speed Controller/2(trq_lim)

== system GVCU_HIL_simscape/Vehicle ==
  note: Signals are Bus signals with 3 values
  Env : Inport
  AxlTrq : Inport  Port=2
  Cmd : Inport  Port=3
  Aerodynamics : Subsystem
  Bus Creator1 : BusCreator  Inputs=3
  Bus Selector : BusSelector  OutputSignals=Ground.G_FL_z,Ground.G_FR_z,Ground.G_RL_z,Ground.G_RR_z  OutputAsBus=on
  Bus Selector1 : BusSelector  OutputSignals=Wind.windx
  Gain : Gain  Gain=3.6
  Memory : Memory
  Memory1 : Memory
  Subsystem : Subsystem
  Subsystem1 : Subsystem  Commented=on
  System Variable Output1 : canoelib/CANoe I//O/System Variable Output  Commented=on  nsName=Checker_Simulink  sysVarName=Force_external  arrayIndex=-1  rawValue=Default  dataType=Default  dataTypeDB=int32  hasEncoding=off  dataTypeCANoe=Get from CANoe
      settings: AttributesFormatString=%<nsName>::%<sysVarName>  SourceProductName=Vector CANoe
  System Variable Output2 : canoelib/CANoe I//O/System Variable Output  Commented=on  nsName=Checker_Simulink  sysVarName=M_extern  arrayIndex=-1  rawValue=Default  dataType=Default  dataTypeDB=int32  hasEncoding=off  dataTypeCANoe=Get from CANoe
      settings: AttributesFormatString=%<nsName>::%<sysVarName>  SourceProductName=Vector CANoe
  Vehicle Body 1DOF Longitudinal : autolibshared/Vehicle Body 1DOF Longitudinal  VariantControl=SL  extFMode=on  extMMode=on  extTamb=off  wind3D=off  aMode=2  NF=2  NR=2  m=veh.mass  a=veh.f  b=veh.r  h=veh.h+(tir.UNLOADED_RADIUSf+tir.UNLOADED_RADIUSr)/2  Cd=veh.aero.CD  Cl=0  Cpm=0  Af=veh.A  x_o=pos.X_0  xdot_o=pos.xdot_0  Pabs=101325  T=273  g=9.81
      settings: LibrarySourceBlock=vehdynlibeom/Vehicle Body 1DOF Longitudinal
  Wheels1 : Subsystem
  to grade : Subsystem
  Veh : Outport
  tag scope: Force_front_wheel=global, Force_rear_wheel=global, Force_wind=global, ModelVel=global, street_steepness=global, wheels=global
  wires:
  Aerodynamics/1(Info) -> Bus Creator1/3  "Aero"
  Vehicle Body 1DOF Longitudinal/1 -> Aerodynamics/1(VehFdbk), Bus Creator1/2  "Body"
  Wheels1/2(FxF) -> [Force_front_wheel], Vehicle Body 1DOF Longitudinal/3  "FxF"
  Wheels1/3(FxR) -> [Force_rear_wheel], Vehicle Body 1DOF Longitudinal/4  "FxR"
  Aerodynamics/2(FAero) -> Vehicle Body 1DOF Longitudinal/1, System Variable Output1/1
  Env/1 -> Bus Selector1/1, Bus Selector/1, Aerodynamics/2(Env)
  Memory1/1 -> Wheels1/5(FzR)
  Bus Selector/1 -> to grade/1(In1)
  Bus Selector1/1 -> [Force_wind], Vehicle Body 1DOF Longitudinal/6  "<windx>"
  Wheels1/1(Wheels) -> [wheels], Bus Creator1/1  "Wheels"
  Memory/1 -> Wheels1/4(FzF)
  to grade/1(Out1) -> [street_steepness], Vehicle Body 1DOF Longitudinal/5
  Aerodynamics/3(MAero) -> Vehicle Body 1DOF Longitudinal/2, System Variable Output2/1
  Vehicle Body 1DOF Longitudinal/3 -> Memory/1
  AxlTrq/1 -> Wheels1/3(AxlTrq)
  Vehicle Body 1DOF Longitudinal/4 -> Memory1/1
  Bus Creator1/1 -> Veh/1  "Vehicle"
  Subsystem/1(Cntrl) -> Wheels1/2(BrkPrs)
  Cmd/1 -> Subsystem/1(Cmd)
  Vehicle Body 1DOF Longitudinal/2 -> Gain/1, Wheels1/1(Vx)  "m/s"
  Gain/1 -> [ModelVel]  "km/h"

== system GVCU_HIL_simscape/Wheel_rates ==
  note: sign is decided by wheel_direction
  meas : Inport
  Abs{,1..3} (4 alike) : Abs  SaturateOnIntegerOverflow=off
  Bus Selector : BusSelector  Commented=on  OutputSignals=Omega
  Bus Selector1 : BusSelector  OutputSignals=vehicle.front.left.tire.omega,vehicle.front.right.tire.omega,vehicle.rear.left.tire.omega,vehicle.rear.right.tire.omega
  Constant{,2..4} (4 alike) : Constant
  Demux : Demux  Commented=on
  From14 : From  Commented=on  GotoTag=wheels
  MATLAB Function2 : MATLAB Function  TreatAsAtomicUnit=on
  Saturation{,1..3} (4 alike) : Saturate  UpperLimit=655.35  LowerLimit=0
  Signal Output : canoelib/CANoe I//O/Signal Output  dbName=dynamic_systems2_bus  nodeName=IEB  msgName=wheel_rates_front  sigName=wheel_rate_fl  rawValue=Default  dataType=Default  dataTypeDB=uint16  hasEncoding=on
      settings: AttributesFormatString=%<sigName>  SourceProductName=Vector CANoe
  Signal Output1 : canoelib/CANoe I//O/Signal Output  dbName=dynamic_systems2_bus  nodeName=IEB  msgName=wheel_rates_front  sigName=wheel_rate_fr  rawValue=Default  dataType=Default  dataTypeDB=uint16  hasEncoding=on
      settings: AttributesFormatString=%<sigName>  SourceProductName=Vector CANoe
  Signal Output10 : canoelib/CANoe I//O/Signal Output  dbName=dynamic_systems2_bus  nodeName=IEB  msgName=wheel_rates_rear  sigName=wheel_direction_rl  rawValue=Default  dataType=Default  dataTypeDB=uint8  hasEncoding=off
      settings: AttributesFormatString=%<sigName>  SourceProductName=Vector CANoe
  Signal Output11 : canoelib/CANoe I//O/Signal Output  dbName=dynamic_systems2_bus  nodeName=IEB  msgName=wheel_rates_rear  sigName=wheel_direction_rr  rawValue=Default  dataType=Default  dataTypeDB=uint8  hasEncoding=off
      settings: AttributesFormatString=%<sigName>  SourceProductName=Vector CANoe
  Signal Output2 : canoelib/CANoe I//O/Signal Output  dbName=dynamic_systems2_bus  nodeName=IEB  msgName=wheel_rates_rear  sigName=wheel_rate_rl  rawValue=Default  dataType=Default  dataTypeDB=uint16  hasEncoding=on
      settings: AttributesFormatString=%<sigName>  SourceProductName=Vector CANoe
  Signal Output3 : canoelib/CANoe I//O/Signal Output  dbName=dynamic_systems2_bus  nodeName=IEB  msgName=wheel_rates_rear  sigName=wheel_rate_rr  rawValue=Default  dataType=Default  dataTypeDB=uint16  hasEncoding=on
      settings: AttributesFormatString=%<sigName>  SourceProductName=Vector CANoe
  Signal Output4 : canoelib/CANoe I//O/Signal Output  dbName=dynamic_systems2_bus  nodeName=IEB  msgName=wheel_rates_front  sigName=wheel_rate_fl_v  rawValue=Default  dataType=Default  dataTypeDB=boolean  hasEncoding=off
      settings: AttributesFormatString=%<sigName>  SourceProductName=Vector CANoe
  Signal Output5 : canoelib/CANoe I//O/Signal Output  dbName=dynamic_systems2_bus  nodeName=IEB  msgName=wheel_rates_front  sigName=wheel_rate_fr_v  rawValue=Default  dataType=Default  dataTypeDB=boolean  hasEncoding=off
      settings: AttributesFormatString=%<sigName>  SourceProductName=Vector CANoe
  Signal Output6 : canoelib/CANoe I//O/Signal Output  dbName=dynamic_systems2_bus  nodeName=IEB  msgName=wheel_rates_rear  sigName=wheel_rate_rl_v  rawValue=Default  dataType=Default  dataTypeDB=boolean  hasEncoding=off
      settings: AttributesFormatString=%<sigName>  SourceProductName=Vector CANoe
  Signal Output7 : canoelib/CANoe I//O/Signal Output  dbName=dynamic_systems2_bus  nodeName=IEB  msgName=wheel_rates_rear  sigName=wheel_rate_rr_v  rawValue=Default  dataType=Default  dataTypeDB=boolean  hasEncoding=off
      settings: AttributesFormatString=%<sigName>  SourceProductName=Vector CANoe
  Signal Output8 : canoelib/CANoe I//O/Signal Output  dbName=dynamic_systems2_bus  nodeName=IEB  msgName=wheel_rates_front  sigName=wheel_direction_fl  rawValue=Default  dataType=Default  dataTypeDB=uint8  hasEncoding=off
      settings: AttributesFormatString=%<sigName>  SourceProductName=Vector CANoe
  Signal Output9 : canoelib/CANoe I//O/Signal Output  dbName=dynamic_systems2_bus  nodeName=IEB  msgName=wheel_rates_front  sigName=wheel_direction_fr  rawValue=Default  dataType=Default  dataTypeDB=uint8  hasEncoding=off
      settings: AttributesFormatString=%<sigName>  SourceProductName=Vector CANoe
  wires:
  Bus Selector1/4 -> MATLAB Function2/1(wheel_rate), Abs3/1  "<omega>"
  Constant4/1 -> Signal Output7/1
  Constant2/1 -> Signal Output5/1
  Constant3/1 -> Signal Output6/1
  Constant/1 -> Signal Output4/1
  MATLAB Function2/1(wheel_direction) -> Signal Output11/1, Signal Output10/1, Signal Output9/1, Signal Output8/1  "refVel"
  Saturation/1 -> Signal Output/1
  Saturation1/1 -> Signal Output1/1
  Saturation2/1 -> Signal Output2/1
  Saturation3/1 -> Signal Output3/1
  Abs/1 -> Saturation/1
  Abs1/1 -> Saturation1/1
  Abs2/1 -> Saturation2/1
  Abs3/1 -> Saturation3/1
  meas/1 -> Bus Selector1/1
  Demux/2 -> ?
  From14/1 -> Bus Selector/1
  Bus Selector/1 -> Demux/1  "<Omega>"
  Demux/3 -> ?
  Bus Selector1/1 -> Abs/1  "<omega>"
  Bus Selector1/3 -> Abs2/1  "<omega>"
  Bus Selector1/2 -> Abs1/1  "<omega>"

== system GVCU_HIL_simscape/clutch control ==
  Bus Creator : BusCreator  Inputs=5
  Bus Creator1 : BusCreator  Inputs=1
  Constant{,1..3} (4 alike) : Constant  Commented=on  Value=5000000
  Constant4 : Constant  Commented=on  Value=0
  control : Outport
  wires:
  Bus Creator/1 -> Bus Creator1/1  "clutch"
  [Center_prs] -> Bus Creator/5  "C"
  [RL_prs] -> Bus Creator/3  "RL"
  [RR_prs] -> Bus Creator/4  "RR"
  [FL_prs] -> Bus Creator/1  "FL"
  [FR_prs] -> Bus Creator/2  "FR"
  Bus Creator1/1 -> control/1

== system GVCU_HIL_simscape/config ==
  " origin" : sm_lib/Body Elements/Spherical Solid  Commented=on  SphereRadius=0.02  SphereRadiusUnits=m  ExportEntireGeometry=off  InertiaType=PointMass  BasedOnType=Density  Density=0  DensityUnits=kg/m^3  Mass=0  MassUnits=kg  CenterOfMass=[0 0 0]  CenterOfMassUnits=m  MomentsOfInertia=[1 1 1]  MomentsOfInertiaUnits=kg*m^2  ProductsOfInertia=[0 0 0]  ProductsOfInertiaUnits=kg*m^2  GraphicType=FromGeometry  MarkerShape=Sphere  MarkerSize=10  GraphicVisPropType=SimpleVisualProperties  GraphicDiffuseColor=[0.0 0.0 0.0]  GraphicOpacity=1  GraphicSpecularColor=[0.5 0.5 0.5 1.0]  GraphicAmbientColor=[0.15 0.15 0.15 1.0]  GraphicEmissiveColor=[0.0 0.0 0.0 1.0]  GraphicShininess=75  DoExposeReferenceFrame=on  SerializedFrames=<Frames/>
  Mechanism Configuration : sm_lib/Utilities/Mechanism Configuration  UniformGravity=Constant  GravityVector=[0 0 -9.80665]  GravityVectorUnits=m/s^2  LinearizationDelta=0.001  JointModeTransitionNonlinearIterations=2
  Solver Configuration : nesl_utility/Solver Configuration  PhysicalDomain=network_engine_domain  SubClassName=solver  LeftPortType=input  RightPortType=generic  Tones=[]  Harmonics=[]  SimulateNoise=off  Profile=off  UseLocalSampling=off  EnableSwitchedLinearOptims=on  FrequencyDomain=off  UseCCode=off  RelTol=0.001  AbsTol=0.001  MinStep=1e-09  ToWorkspace=off  RevertToSquareIcSolve=off  NumHomotopyIterations=100  PhasorMode=off  PhasorModeNumHarmonics=1  ConsistencySolver=NEWTON_XTOL_AFTER_FTOL  CanonicalOrdering=UNORDERED  OptimizeIntermediates=UNOPTIMIZED  IndexReductionMethod=DerivativeReplacement  DoDC=off  ResidualTolerance=1e-09  ConsistencyTolSource=GLOBAL  ConsistencyAbsTol=0.001  ConsistencyRelTol=0.001  ConsistencyTolFactor=0.001  UseLocalSolver=on  LocalSolverChoice=NE_BACKWARD_EULER_ADVANCER  ResolveIndetEquations=on  FunctionEvalNumThread=1  LocalSolverSampleTime=0.002  DoFixedCost=on  MaxNonlinIter=3  MaxModeIter=2  ComputeImpulses=off  ImpulseIterations=2  LinearAlgebra=auto  LinearAlgebraNumThread=0  EquationFormulation=NE_TIME_EF  DelaysMemoryBudget=1024  AutomaticFiltering=on  FilteringTimeConstant=0.001  PartitionStorageMethod=AS_NEEDED  PartitionMemoryBudget=1024  PartitionMethod=ROBUST  MultibodyUseLocalSolver=off  MultibodyLocalSolverChoice=ODE3  MultibodyLocalSolverSampleTime=0.001
  World Frame : sm_lib/Frames and Transforms/World Frame
  ref : PMIOPort  Side=Right
  connections:
  Mechanism Configuration/RConn1 -- Solver Configuration/RConn1 -- World Frame/RConn1 -- " origin"/RConn1 -- ref/RConn1

== system GVCU_HIL_simscape/friction ==
  Bus Creator{,1..3} (4 alike) : BusCreator  Inputs=2
  Bus Creator4 : BusCreator  Inputs=4
  Constant : Constant  Value=front.wheel.magic_param.SCALING_COEFFICIENTS.LMUX
  Constant1 : Constant  Value=front.wheel.magic_param.SCALING_COEFFICIENTS.LMUY
  Constant2 : Constant  Value=front.wheel.magic_param.SCALING_COEFFICIENTS.LMUX
  Constant3 : Constant  Value=front.wheel.magic_param.SCALING_COEFFICIENTS.LMUY
  Constant4 : Constant  Value=rear.wheel.magic_param.SCALING_COEFFICIENTS.LMUX
  Constant5 : Constant  Value=rear.wheel.magic_param.SCALING_COEFFICIENTS.LMUY
  Constant6 : Constant  Value=rear.wheel.magic_param.SCALING_COEFFICIENTS.LMUX
  Constant7 : Constant  Value=rear.wheel.magic_param.SCALING_COEFFICIENTS.LMUY
  friction : Outport
  wires:
  Constant/1 -> Bus Creator/1  "front_left_lmux"
  Constant1/1 -> Bus Creator/2  "front_left_lmuy"
  Constant2/1 -> Bus Creator1/1  "front_right_lmux"
  Constant3/1 -> Bus Creator1/2  "front_right_lmuy"
  Constant4/1 -> Bus Creator3/1  "rear_left_lmux"
  Constant5/1 -> Bus Creator3/2  "rear_left_lmuy"
  Constant6/1 -> Bus Creator2/1  "rear_right_lmux"
  Constant7/1 -> Bus Creator2/2  "rear_right_lmuy"
  Bus Creator2/1 -> Bus Creator4/4  "RR"
  Bus Creator3/1 -> Bus Creator4/3  "RL"
  Bus Creator4/1 -> friction/1
  Bus Creator1/1 -> Bus Creator4/2  "FR"
  Bus Creator/1 -> Bus Creator4/1  "FL"

== system GVCU_HIL_simscape/ground ==
  airfield : Subsystem
  ref : PMIOPort  Side=Left
  connections:
  airfield/LConn1 -- ref/RConn1
